simulink model "SSmodel_LQ_regulator"  (Simulink 7.5)
settings: Solver=ode45  StartTime=0.0  StopTime=10  FixedStep=Ts  MaxStep=1e-2  RelTol=1e-3
values from neighbouring files (symbols this model uses):
  Xl0 = [0.03;0]    [TSC160127ProvaMatlab.m]
undefined symbols (not defined in the file or in its folder): A, B, C, K
settings Model: Creator=lbiagiotti  LastModifiedBy=Biagio
settings DebuggingCC: SaveWithParameterizedLinksMsg=none  StrictBusMsg=Warning
settings HardwareCC: TargetHWDeviceType=32-bit Generic
settings GRTTargetCC: TargetFcnLib=ansi_tfl_tmw.mat

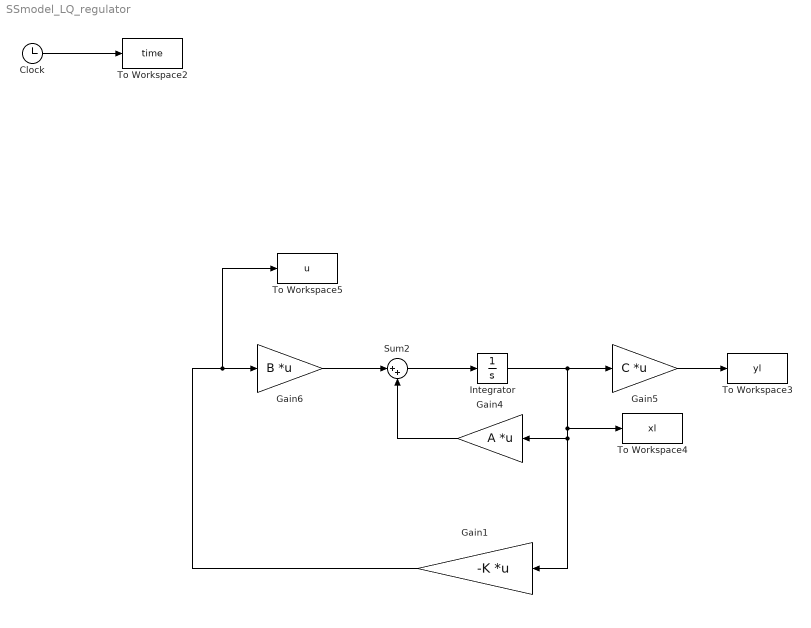
== system SSmodel_LQ_regulator ==
  Clock : Clock
      settings: Decimation=10
  Gain1 : Gain  Gain=-K  Multiplication=Matrix(K*u)  ParameterDataType=sfix(16)  ParameterScaling=2^0  OutDataType=sfix(16)  OutScaling=2^0
  Gain4 : Gain  Gain=A  Multiplication=Matrix(K*u)  ParameterDataType=sfix(16)  ParameterScaling=2^0  OutDataType=sfix(16)  OutScaling=2^0
  Gain5 : Gain  Gain=C  Multiplication=Matrix(K*u)  ParameterDataType=sfix(16)  ParameterScaling=2^0  OutDataType=sfix(16)  OutScaling=2^0
  Gain6 : Gain  Gain=B  Multiplication=Matrix(K*u)  ParameterDataType=sfix(16)  ParameterScaling=2^0  OutDataType=sfix(16)  OutScaling=2^0
  Integrator : Integrator  InitialCondition=Xl0
  Sum2 : Sum  Inputs=|++  OutDataType=sfix(16)  OutScaling=2^0
  To Workspace2 : ToWorkspace  VariableName=time  SampleTime=-1  SaveFormat=Array
  To Workspace3 : ToWorkspace  VariableName=yl  SampleTime=-1  SaveFormat=Array
  To Workspace4 : ToWorkspace  VariableName=xl  SampleTime=-1  SaveFormat=Array
  To Workspace5 : ToWorkspace  VariableName=u  SampleTime=-1  SaveFormat=Array
  wires:
  Gain6/1 -> Sum2/1
  Gain4/1 -> Sum2/2
  Sum2/1 -> Integrator/1
  Integrator/1 -> To Workspace4/1, Gain4/1, Gain1/1, Gain5/1
  Gain5/1 -> To Workspace3/1
  Clock/1 -> To Workspace2/1
  Gain1/1 -> Gain6/1, To Workspace5/1
